simulink library "INT_InjCrv_PoI2"  (R2016b)
settings: Solver=VariableStepAuto  StartTime=0.0  StopTime=10.0  RelTol=1e-3
settings Model: Creator=Wei Liang  LastModifiedBy=Wei Liang

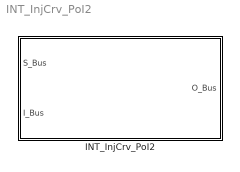
== system INT_InjCrv_PoI2 ==
  INT_InjCrv_PoI2 : Subsystem

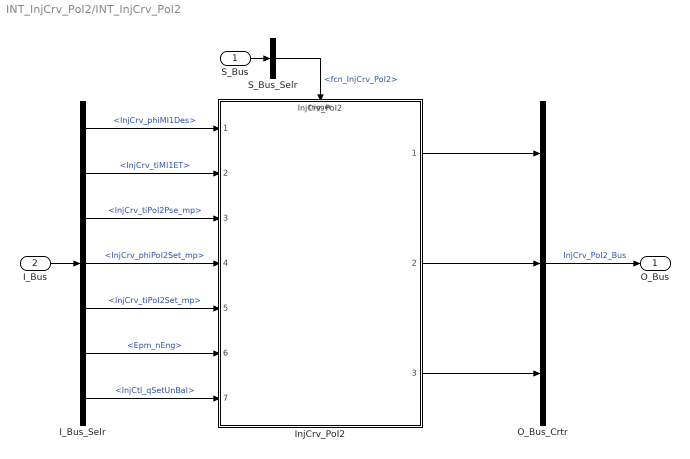
== system INT_InjCrv_PoI2/INT_InjCrv_PoI2 ==
  S_Bus : Inport
  I_Bus : Inport  Port=2
  I_Bus_Selr : BusSelector  OutputSignals=InjCrv_phiMI1Des,InjCrv_tiMI1ET,InjCrv_tiPoI2Pse_mp,InjCrv_phiPoI2Set_mp,InjCrv_tiPoI2Set_mp,Epm_nEng,InjCtl_qSetUnBal
  InjCrv_PoI2 : ModelReference  ModelNameDialog=InjCrv_PoI2  SimulationMode=Normal  ModelReferenceVersion=1.22  TriggerPortName=function  TriggerPortTriggerType=function-call  TriggerPortStatesWhenEnabling=held
  O_Bus_Crtr : BusCreator  Inputs=3
  S_Bus_Selr : BusSelector  OutputSignals=fcn_InjCrv_PoI2
  O_Bus : Outport
  wires:
  S_Bus_Selr/1 -> InjCrv_PoI2/Trigger  "<fcn_InjCrv_PoI2>"
  S_Bus/1 -> S_Bus_Selr/1
  I_Bus/1 -> I_Bus_Selr/1
  I_Bus_Selr/1 -> InjCrv_PoI2/1  "<InjCrv_phiMI1Des>"
  I_Bus_Selr/2 -> InjCrv_PoI2/2  "<InjCrv_tiMI1ET>"
  I_Bus_Selr/3 -> InjCrv_PoI2/3  "<InjCrv_tiPoI2Pse_mp>"
  I_Bus_Selr/4 -> InjCrv_PoI2/4  "<InjCrv_phiPoI2Set_mp>"
  I_Bus_Selr/5 -> InjCrv_PoI2/5  "<InjCrv_tiPoI2Set_mp>"
  I_Bus_Selr/6 -> InjCrv_PoI2/6  "<Epm_nEng>"
  I_Bus_Selr/7 -> InjCrv_PoI2/7  "<InjCtl_qSetUnBal>"
  O_Bus_Crtr/1 -> O_Bus/1  "InjCrv_PoI2_Bus"
  InjCrv_PoI2/1 -> O_Bus_Crtr/1
  InjCrv_PoI2/2 -> O_Bus_Crtr/2
  InjCrv_PoI2/3 -> O_Bus_Crtr/3
